simulink model "sfcndemo_stspace"  (Simulink 6.0)
settings: Solver=ode3  StartTime=0.0  StopTime=10.0  RelTol=1e-3
settings Model: Creator=The MathWorks Inc.  LastModifiedBy=batserve  ExtModeTrigMode=oneshot  ExtModeArmWhenConnect=off  ExtModeAutoUpdateStatusClock=off
settings DataIOCC: LimitDataPoints=off
settings OptimizationCC: BooleanDataType=off
settings DebuggingCC: CheckExecutionContextPreStartOutputMsg=on  CheckExecutionContextRuntimeOutputMsg=on  SolverPrmCheckMsg=none
settings HardwareCC: TargetUnknown=on

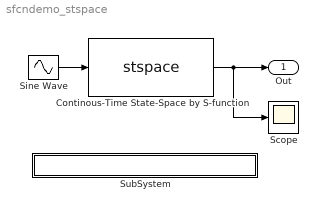
== system sfcndemo_stspace ==
  Continous-Time State-Space by S-function : S-Function  FunctionName=stspace  Parameters=a,b,c,d,x0  mask(S-function: stspace){a=[-0.09 -0.01; 1 0], b=[1 -7; 0 -2], c=[0 2; 1 -5], d=[-3 0; 1 0], x0=[]}
      mask prompts: x0 "Initial condition:"
      mask help: This is a S-function block which is the state-space system with dynamic inputs, outputs and states.
      mask Display: disp('dx/dt = A*X + B*U\n Y      = C*X + D*U ');
  Scope : Scope
      settings: TimeRange=10  YMin=-200  YMax=500
  Sine Wave : Sin  Amplitude=[1 2]  SampleTime=0
  SubSystem : Subsystem  PropExecContextAcrossSSBoundary=on
      settings: OpenFcn=edit(fullfile(matlabroot,'simulink','src','stspace.c'))
      mask Display: disp('matlabroot\simulink\src\stspace.c');
  Out : Outport  InitialOutput=0
  wires:
  Sine Wave/1 -> Continous-Time State-Space by S-function/1
  Continous-Time State-Space by S-function/1 -> Out/1, Scope/1

== system sfcndemo_stspace/SubSystem ==
